simulink model "nonlineare_1_sim"  (Simulink 6.0)
settings: Solver=ode45  StartTime=0.0  StopTime=2  RelTol=1e-3
libraries: simulink x1
settings Model: LastModifiedBy=enrico
settings DataIOCC: SaveOutput=off  SaveTime=off
settings OptimizationCC: BooleanDataType=off
settings DebuggingCC: SolverPrmCheckMsg=none
settings HardwareCC: TargetUnknown=on
settings GRTTargetCC: ModelReferenceCompliant=off  MatFileLogging=off

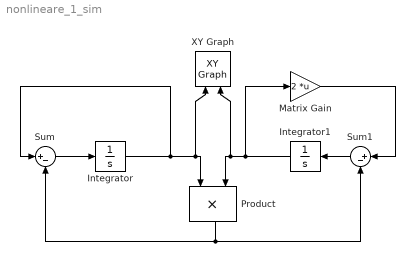
== system nonlineare_1_sim ==
  Integrator : Integrator  InitialCondition=10
  Integrator1 : Integrator  Orientation=left  InitialCondition=10
  Matrix Gain : Gain  Gain=2  Multiplication=Matrix(K*u)  SaturateOnIntegerOverflow=on
  Product : Product  Orientation=down  SaturateOnIntegerOverflow=on  RndMeth=Zero  InputSameDT=on
  Sum : Sum  Inputs=|+-  SaturateOnIntegerOverflow=on  InputSameDT=on
  Sum1 : Sum  Orientation=left  Inputs=|+-  SaturateOnIntegerOverflow=on  InputSameDT=on
  XY Graph : simulink/Sinks/XY Graph  Orientation=up  xmin=-20  xmax=20  ymin=-20  ymax=20  st=-1
  wires:
  Integrator/1 -> Sum/1, Product/1, XY Graph/1
  Integrator1/1 -> Matrix Gain/1, Product/2, XY Graph/2
  Sum/1 -> Integrator/1
  Product/1 -> Sum/2, Sum1/2
  Matrix Gain/1 -> Sum1/1
  Sum1/1 -> Integrator1/1
